simulink model "Boat_model_joystick"  (Simulink 6.6)
settings: Solver=ode3  StartTime=0.0  StopTime=10000.0  FixedStep=1  RelTol=1e-3
libraries: simulink x2, vrlib x1
settings Model: Creator=Administrator  LastModifiedBy=Administrator

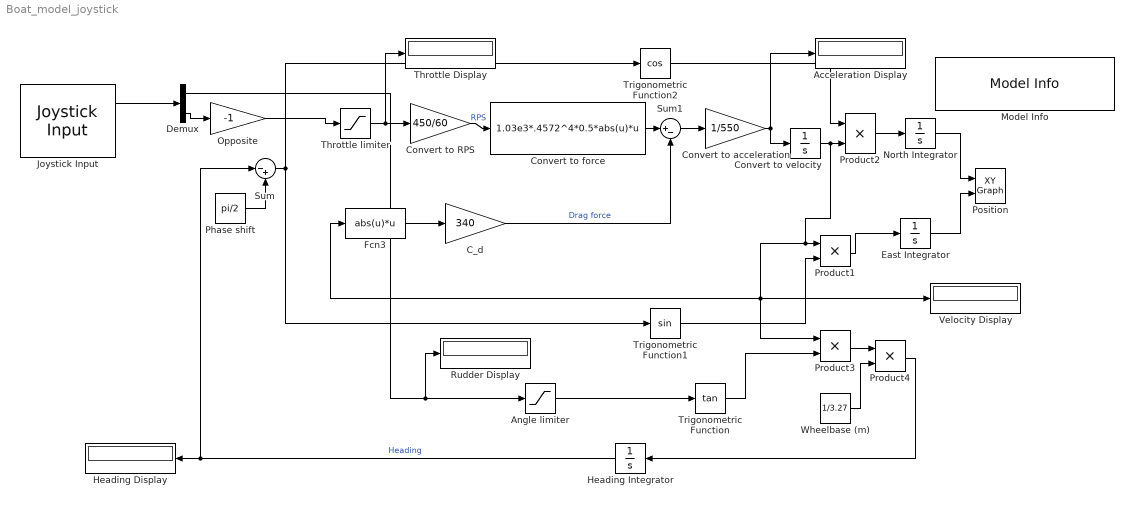
== system Boat_model_joystick ==
  Acceleration Display : Display
  Angle limiter : Saturate  UpperLimit=1  LowerLimit=-1
  C_d : Gain  Gain=340
  Convert to RPS : Gain  Gain=450/60
  Convert to acceleration : Gain  Gain=1/550
  Convert to force : Fcn  Expr=1.03e3*.4572^4*0.5*abs(u)*u
  Convert to velocity : Integrator
  Demux : Demux  Outputs=3
  East Integrator : Integrator
  Fcn3 : Fcn  Expr=abs(u)*u
  Heading Display : Display
  Heading Integrator : Integrator  Orientation=left
  Joystick Input : vrlib/Joystick Input  joyid=1  adjustports=on  forcefeed=off
  Model Info : simulink/Model-Wide Utilities/Model Info  SystemSampleTime=-1  InitialBlockCM=None  BlockCM=None  Frame=on  DisplayStringWithTags=|  HorizontalTextAlignment=Center  LeftAlignmentValue=0.5  SourceBlockDiagram=Boat_model_joystick  TagMaxNumber=20
      | Kinematic model of the autoboat.
      | Version %<ModelVersion>
  North Integrator : Integrator
  Opposite : Gain  Gain=-1
  Phase shift : Constant  Value=pi/2
  Position : simulink/Sinks/XY Graph  SystemSampleTime=-1  xmin=-10000  xmax=10000  ymin=-10000  ymax=10000  st=-1
  Product{1..4} (4 alike) : Product  RndMeth=Zero
  Rudder Display : Display
  Sum : Sum  Inputs=|-+
  Sum1 : Sum  Inputs=|+-
  Throttle Display : Display
  Throttle limiter : Saturate  UpperLimit=1  LowerLimit=0
  Trigonometric Function : Trigonometry  Operator=tan  OutputSignalType=real
  Trigonometric Function1 : Trigonometry  OutputSignalType=real
  Trigonometric Function2 : Trigonometry  Operator=cos  OutputSignalType=real
  Velocity Display : Display
  Wheelbase (m) : Constant  Value=1/3.27
  wires:
  North Integrator/1 -> Position/1
  Trigonometric Function2/1 -> Product2/1
  East Integrator/1 -> Position/2
  Trigonometric Function1/1 -> Product1/2
  Product2/1 -> North Integrator/1
  Trigonometric Function/1 -> Product3/2
  Product3/1 -> Product4/1
  Sum/1 -> Trigonometric Function1/1, Trigonometric Function2/1
  Phase shift/1 -> Sum/2
  Product1/1 -> East Integrator/1
  Angle limiter/1 -> Trigonometric Function/1
  Product4/1 -> Heading Integrator/1
  Throttle limiter/1 -> Convert to RPS/1, Throttle Display/1
  Convert to RPS/1 -> Convert to force/1  "RPS"
  Convert to velocity/1 -> Product2/2, Product1/1, Product3/1, Fcn3/1, Velocity Display/1
  Fcn3/1 -> C_d/1
  C_d/1 -> Sum1/2  "Drag force"
  Convert to acceleration/1 -> Convert to velocity/1, Acceleration Display/1
  Sum1/1 -> Convert to acceleration/1
  Convert to force/1 -> Sum1/1
  Joystick Input/1 -> Demux/1
  Demux/1 -> Angle limiter/1, Rudder Display/1
  Opposite/1 -> Throttle limiter/1
  Demux/3 -> Opposite/1
  Heading Integrator/1 -> Heading Display/1, Sum/1  "Heading"
  Wheelbase (m)/1 -> Product4/2
